simulink model "Test_newPR9July"  (R2022b)
settings: Solver=VariableStepAuto  StartTime=0.0  StopTime=25  RelTol=1e-3
values from neighbouring files (symbols this model uses):
  C_f = 0.000112315*9    (= 0.001010835)    [Main.m]    (also in PSO_2paras.m = swarm(i,2); PSO_filter_2paras.m = swarm(i,2)/10000; Primary_test1.m; Script_18June.m = 0.0112315)
  f_c = 50e3    (= 50000)    [Main.m]    (also in Primary_test1.m; Script_18June.m; Script_23June.m; Script_5thJune.m)
  k = -0.5    [Main.m]    (also in Primary_test1.m; Savedata.m = 0.2909; Script_18June.m = 0.5; Script_23June.m)
  K_h11 = 0    [Main.m]    (also in PSO_HC.m = swarm(i,4); Primary_test1.m; Script_18June.m; Script_23June.m)
  K_h13 = 0    [Main.m]    (also in Primary_test1.m; Script_18June.m; Script_23June.m; Script_5thJune.m)
  K_h5 = 0    [Main.m]    (also in PSO_HC.m = swarm(i,1); Primary_test1.m = 1; Script_18June.m; Script_23June.m)
  K_h7 = 0    [Main.m]    (also in PSO_HC.m = swarm(i,2); Primary_test1.m; Script_18June.m; Script_23June.m)
  K_h9 = 0    [Main.m]    (also in PSO_HC.m = swarm(i,3); Script_18June.m; Script_23June.m; Script_5thJune.m)
  ki_pr = 160    [Main.m]    (also in PSO.m = swarm(i,2); Primary_test1.m; Savedata.m = 422.4716; Script_18June.m = 150)
  kL = 1e-7    (= 1e-07)    [Main.m]    (also in Primary_test1.m; Script_18June.m; Script_23June.m; Script_5thJune.m)
  Kp_pr = 1.7    [Main.m]    (also in PSO.m = swarm(i,1); Primary_test1.m; Savedata.m = 0.9028; Script_18June.m = 1)
  L_f = 0.000659829*1.4    (= 0.0009237606)    [Main.m]    (also in PSO_2paras.m = swarm(i,1); PSO_filter_2paras.m = swarm(i,1); Primary_test1.m; Script_18June.m = 0.000295603392)
  L_in1 = 0.35e-3    (= 0.00035)    [Main.m]    (also in Primary_test1.m; Script_18June.m; Script_23June.m; Script_5thJune.m)
  L_in2 = 0.35e-3    (= 0.00035)    [Main.m]    (also in Primary_test1.m; Script_18June.m; Script_23June.m; Script_5thJune.m)
  LD_ref1 = 100e-6    (= 0.0001)    [Main.m]    (also in Primary_test1.m; Script_18June.m = 5e-05; Script_23June.m = 1e-05; Script_5thJune.m = 1e-05)
  lo_co = 0.1    [Main.m]    (also in Primary_test1.m; Script_18June.m; Script_23June.m; Script_5thJune.m)
  load_off = 28    [Main.m]    (also in Primary_test1.m = 2; Script_18June.m; Script_23June.m; Script_5thJune.m = 10)
  load_on = 0.21    [Main.m]    (also in Primary_test1.m = 1; Script_18June.m; Script_23June.m; Script_5thJune.m)
  m_p1 = 9.4e-5/droopDivide    (= 9.4e-06)    [Main.m]    (also in Primary_test1.m; Script_18June.m = 9.4e-05; Script_23June.m = 9.4e-05; Script_5thJune.m = 5e-05)
  m_p2 = 9.4e-5/droopDivide    (= 9.4e-06)    [Main.m]    (also in Primary_test1.m; Script_18June.m = 9.4e-05; Script_23June.m = 9.4e-05; Script_5thJune.m = 5e-05)
  m_p3 = 11.4e-5/droopDivide    (= 1.14e-05)    [Main.m]    (also in Primary_test1.m; Script_18June.m = 0.000114; Script_23June.m = 0.000114; Script_5thJune.m = 6.42857142857e-05)
  m_p4 = 11.4e-5/droopDivide    (= 1.14e-05)    [Main.m]    (also in Primary_test1.m; Script_18June.m = 0.000114; Script_23June.m = 0.000114; Script_5thJune.m = 6.42857142857e-05)
  n_q1 = 1.3e-3/droopDivide2    (= 6.5e-05)    [Main.m]    (also in Primary_test1.m; Script_18June.m; Script_23June.m; Script_5thJune.m = 0.2)
  n_q2 = 1.3e-3/droopDivide2    (= 6.5e-05)    [Main.m]    (also in Primary_test1.m; Script_18June.m; Script_23June.m; Script_5thJune.m = 0.2)
  n_q3 = 1.5e-3/droopDivide2    (= 7.5e-05)    [Main.m]    (also in Primary_test1.m; Script_18June.m; Script_23June.m; Script_5thJune.m = 0.257142857143)
  n_q4 = 1.5e-3/droopDivide2    (= 7.5e-05)    [Main.m]    (also in Primary_test1.m; Script_18June.m; Script_23June.m; Script_5thJune.m = 0.257142857143)
  PMW = V_nom/0.55    [Main.m]    (also in Primary_test1.m; Script_18June.m = V_nom/0.4; Script_23June.m; Script_5thJune.m = 220*sqrt(2))
  R_f = 0.35    [Main.m]    (also in PSO_filter_2paras.m = 10*L_f; Primary_test1.m; Savedata.m = 0.249593207053; Script_18June.m = 0.1)
  R_in1 = 0.03    [Main.m]    (also in Primary_test1.m; Script_18June.m; Script_23June.m; Script_5thJune.m)
  R_in2 = 0.03    [Main.m]    (also in Primary_test1.m; Script_18June.m; Script_23June.m; Script_5thJune.m)
  Ts = 10e-6    (= 1e-05)    [Main.m]    (also in Primary_test1.m; Script_18June.m; Script_23June.m; Script_5thJune.m)
  V_nom = 220*sqrt(2)    [Main.m]    (also in Primary_test1.m; Script_18June.m; Script_23June.m; Script_5thJune.m)
  Vdc = 600    [Main.m]    (also in Primary_test1.m; Script_18June.m; Script_23June.m; Script_5thJune.m)
  w_c_high = 2*pi*50    (= 314.159265359)    [Main.m]    (also in Primary_test1.m; Script_18June.m = 307.876080052; Script_23June.m; Script_5thJune.m = 307.876080052)
  w_nom = 2*pi*f    (= 314.159265359)    [Main.m]    (also in Primary_test1.m; Script_18June.m; Script_23June.m; Script_5thJune.m)
  wc_hc = 1    [Main.m]    (also in Primary_test1.m; Script_18June.m = 0.3; Script_23June.m; Script_5thJune.m = 0.3)
  wc_pr = 3    [Main.m]    (also in PSO.m = swarm(i,3); Primary_test1.m; Savedata.m = 1.36672; Script_18June.m = 1.5)
undefined symbols (not defined in the file or in its folder): i
libraries: eeGeneralControl x16, spsThreePhaseSeriesRLCBranchLib x15, spsThreePhaseVIMeasurementLib x12, spsabctodq0Lib x12, spsabctoAlphaBetaZeroLib x9, slpidlib x8, spsThreePhaseSeriesRLCLoadLib x6, spsThreePhaseBreakerLib x6, spsDCVoltageSourceLib x5, spsSeriesRLCBranchLib x5, spsTriangleGeneratorLib x4, spsTwoLevelConverterLib x4
(part 4 of 4)

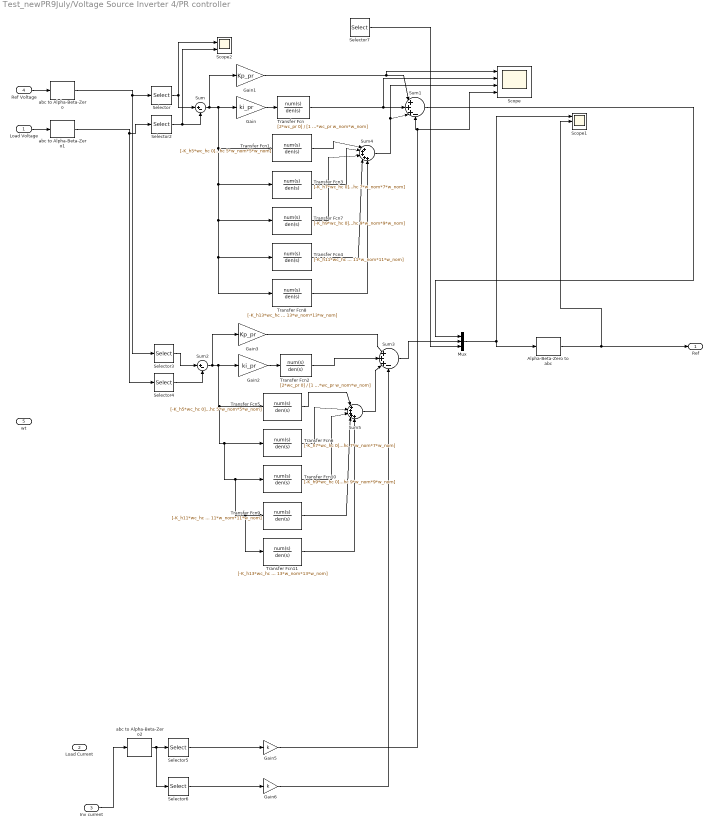
== system Test_newPR9July/Voltage Source Inverter 4/PR controller ==
  Load Voltage : Inport
  Load Current : Inport  Port=2
  Inv current : Inport  Port=3
  Ref Voltage : Inport  Port=4
  wt : Inport  Port=5
  Alpha-Beta-Zero to abc : spsAlphaBetaZerotoabcLib/Alpha-Beta-Zero to abc
      settings: LibrarySourceBlock=|
      | sps_lib/Control/Alpha-Beta-Zero
      | to abc
  Gain : Gain  Gain=ki_pr
  Gain1 : Gain  Gain=Kp_pr
  Gain2 : Gain  Gain=ki_pr
  Gain3 : Gain  Gain=Kp_pr
  Gain5 : Gain  Gain=k
  Gain6 : Gain  Gain=k
  Mux : Mux  Inputs=3
  Scope : Scope  NumInputPorts=4
  Scope1 : Scope  NumInputPorts=3
  Scope2 : Scope  NumInputPorts=2
  Selector : Selector  InputPortWidth=3  IndexOptions=Index vector (dialog)  Indices=[1]  OutputSizes=1
  Selector2 : Selector  InputPortWidth=3  IndexOptions=Index vector (dialog)  Indices=[1]  OutputSizes=1
  Selector3 : Selector  InputPortWidth=3  IndexOptions=Index vector (dialog)  Indices=[2]  OutputSizes=1
  Selector4 : Selector  InputPortWidth=3  IndexOptions=Index vector (dialog)  Indices=[2]  OutputSizes=1
  Selector5 : Selector  InputPortWidth=3  IndexOptions=Index vector (dialog)  Indices=[1]  OutputSizes=1
  Selector6 : Selector  InputPortWidth=3  IndexOptions=Index vector (dialog)  Indices=[2]  OutputSizes=1
  Selector7 : Selector  InputPortWidth=3  IndexOptions=Index vector (dialog)  Indices=[3]  OutputSizes=1
  Sum : Sum  Inputs=|+-
  Sum1 : Sum  Inputs=|+++-
  Sum2 : Sum  Inputs=|+-
  Sum3 : Sum  Inputs=|+++-
  Sum4 : Sum  Inputs=|+++++
  Sum5 : Sum  Inputs=|+++++
  Transfer Fcn : TransferFcn  Numerator=[2*wc_pr 0]  Denominator=[1 2*wc_pr*wc_pr w_nom*w_nom]
  Transfer Fcn1 : TransferFcn  Numerator=[-K_h5*wc_hc 0]  Denominator=[1 2*wc_hc 5*w_nom*5*w_nom]
  Transfer Fcn10 : TransferFcn  Numerator=[-K_h9*wc_hc 0]  Denominator=[1 2*wc_hc 9*w_nom*9*w_nom]
  Transfer Fcn11 : TransferFcn  Numerator=[-K_h13*wc_hc 0]  Denominator=[1 2*wc_hc 13*w_nom*13*w_nom]
  Transfer Fcn2 : TransferFcn  Numerator=[2*wc_pr 0]  Denominator=[1 2*wc_pr*wc_pr w_nom*w_nom]
  Transfer Fcn3 : TransferFcn  Numerator=[-K_h7*wc_hc 0]  Denominator=[1 2*wc_hc 7*w_nom*7*w_nom]
  Transfer Fcn4 : TransferFcn  Numerator=[-K_h11*wc_hc 0]  Denominator=[1 2*wc_hc 11*w_nom*11*w_nom]
  Transfer Fcn5 : TransferFcn  Numerator=[-K_h5*wc_hc 0]  Denominator=[1 2*wc_hc 5*w_nom*5*w_nom]
  Transfer Fcn6 : TransferFcn  Numerator=[-K_h7*wc_hc 0]  Denominator=[1 2*wc_hc 7*w_nom*7*w_nom]
  Transfer Fcn7 : TransferFcn  Numerator=[-K_h9*wc_hc 0]  Denominator=[1 2*wc_hc 9*w_nom*9*w_nom]
  Transfer Fcn8 : TransferFcn  Numerator=[-K_h13*wc_hc 0]  Denominator=[1 2*wc_hc 13*w_nom*13*w_nom]
  Transfer Fcn9 : TransferFcn  Numerator=[-K_h11*wc_hc 0]  Denominator=[1 2*wc_hc 11*w_nom*11*w_nom]
  abc to Alpha-Beta-Zero : spsabctoAlphaBetaZeroLib/abc to Alpha-Beta-Zero
  abc to Alpha-Beta-Zero1 : spsabctoAlphaBetaZeroLib/abc to Alpha-Beta-Zero
  abc to Alpha-Beta-Zero2 : spsabctoAlphaBetaZeroLib/abc to Alpha-Beta-Zero
  Ref : Outport
  wires:
  Ref Voltage/1 -> abc to Alpha-Beta-Zero/1
  Selector/1 -> Sum/1, Scope2/1
  Selector2/1 -> Sum/2, Scope2/2
  Sum/1 -> Gain1/1, Transfer Fcn8/1, Transfer Fcn4/1, Transfer Fcn7/1, Transfer Fcn3/1, Transfer Fcn1/1, Gain/1
  Gain/1 -> Transfer Fcn/1
  Gain1/1 -> Sum1/1, Scope/1
  Transfer Fcn/1 -> Scope/2, Sum1/2
  Sum2/1 -> Gain3/1, Transfer Fcn11/1, Transfer Fcn9/1, Transfer Fcn10/1, Transfer Fcn6/1, Transfer Fcn5/1, Gain2/1
  Selector3/1 -> Sum2/1
  Gain2/1 -> Transfer Fcn2/1
  Transfer Fcn2/1 -> Sum3/2
  Gain3/1 -> Sum3/1
  abc to Alpha-Beta-Zero2/1 -> Selector6/1, Selector5/1
  Sum1/1 -> Mux/1
  Sum3/1 -> Mux/2
  Mux/1 -> Alpha-Beta-Zero to abc/1, Scope1/1
  Inv current/1 -> abc to Alpha-Beta-Zero2/1
  Sum4/1 -> Sum1/3, Scope/3
  Transfer Fcn1/1 -> Sum4/1
  Transfer Fcn3/1 -> Sum4/2
  Transfer Fcn6/1 -> Sum5/2
  Selector4/1 -> Sum2/2
  Sum5/1 -> Sum3/3
  Transfer Fcn7/1 -> Sum4/3
  Transfer Fcn4/1 -> Sum4/4
  Transfer Fcn8/1 -> Sum4/5
  Transfer Fcn10/1 -> Sum5/3
  Transfer Fcn9/1 -> Sum5/4
  Transfer Fcn11/1 -> Sum5/5
  Selector6/1 -> Gain6/1
  Selector5/1 -> Gain5/1
  Transfer Fcn5/1 -> Sum5/1
  Selector7/1 -> Mux/3
  Gain5/1 -> Sum1/4, Scope/4
  Gain6/1 -> Sum3/4
  Load Voltage/1 -> abc to Alpha-Beta-Zero1/1
  abc to Alpha-Beta-Zero/1 -> Selector3/1, Selector/1
  abc to Alpha-Beta-Zero1/1 -> Selector4/1, Selector2/1
  Alpha-Beta-Zero to abc/1 -> Scope1/2, Ref/1

== system Test_newPR9July/Voltage Source Inverter 4/dq converter ==
  Vodq : Inport
  Iodq : Inport  Port=2
  Ildq : Inport  Port=3
  wt : Inport  Port=4
  Scope : Scope
  Scope1 : Scope
  Subsystem : Subsystem
  Subsystem1 : Subsystem
  Subsystem2 : Subsystem
  Vod : Outport
  Voq : Outport  Port=2
  Iod : Outport  Port=3
  Ioq : Outport  Port=4
  Ild : Outport  Port=5
  Ilq : Outport  Port=6
  wires:
  Subsystem/1(Out1) -> Scope/1, Vod/1  "Vod"
  Subsystem1/1(Out1) -> Iod/1  "Iod"
  Subsystem/2(Out2) -> Voq/1  "Voq"
  wt/1 -> Subsystem2/2(wt), Subsystem1/2(wt), Subsystem/2(wt)
  Subsystem1/2(Out2) -> Ioq/1  "Ioq"
  Iodq/1 -> Subsystem1/1(abc)
  Subsystem2/2(Out2) -> Ilq/1  "Ilq"
  Ildq/1 -> Subsystem2/1(abc)
  Vodq/1 -> Subsystem/1(abc)
  Subsystem2/1(Out1) -> Scope1/1, Ild/1  "Vod"

== system Test_newPR9July/Voltage Source Inverter 1/PLL_1p1/TienXuly ==
  v : Inport
  Gain : Gain  Gain=k
  Integrator : Integrator
  Integrator1 : Integrator
  Locthongthap : TransferFcn  Denominator=[1/fc2 1]
  Mux : Mux  Inputs=2
  Product : Product  RndMeth=Zero
  Product1 : Product  RndMeth=Zero
  Sum : Sum  Inputs=|+-
  Sum1 : Sum  Inputs=|+-
  Sum2 : Sum  Inputs=|+-
  v'-qv' : Scope
  wloc : Constant  Value=fc1*2*pi
  v' : Outport  VectorParamsAs1DForOutWhenUnconnected=off
  v'q : Outport  Port=2  VectorParamsAs1DForOutWhenUnconnected=off
  wires:
  Sum/1 -> Gain/1
  Gain/1 -> Sum1/1, Locthongthap/1
  Sum1/1 -> Product/1
  wloc/1 -> Product/2, Product1/1
  Product/1 -> Integrator/1
  Product1/1 -> Integrator1/1
  Integrator1/1 -> Sum1/2, Sum2/1
  Integrator/1 -> Product1/2, Sum/2, Mux/2, v'/1
  Locthongthap/1 -> Sum2/2
  v/1 -> Sum/1
  Sum2/1 -> v'q/1, Mux/1
  Mux/1 -> v'-qv'/1

== system Test_newPR9July/Voltage Source Inverter 1/PLL_1p1/apha-beta=>dq ==
  Theta : Inport
  Uapha : Inport  Port=2
  Ubeta : Inport  Port=3
  Mux : Mux  Inputs=3
  Tinhvd : Fcn  Expr=(u[2]*cos(u[1])+u[3]*sin(u[1]))
  Tinhvq : Fcn  Expr=(-u[2]*sin(u[1])+u[3]*cos(u[1]))
  vq : Outport  VectorParamsAs1DForOutWhenUnconnected=off
  vd : Outport  Port=2  VectorParamsAs1DForOutWhenUnconnected=off
  wires:
  Theta/1 -> Mux/1
  Uapha/1 -> Mux/2
  Ubeta/1 -> Mux/3
  Mux/1 -> Tinhvd/1, Tinhvq/1
  Tinhvd/1 -> vd/1
  Tinhvq/1 -> vq/1

== system Test_newPR9July/Voltage Source Inverter 1/PLL_1p2/TienXuly ==
  v : Inport
  Gain : Gain  Gain=k
  Integrator : Integrator
  Integrator1 : Integrator
  Locthongthap : TransferFcn  Denominator=[1/fc2 1]
  Mux : Mux  Inputs=2
  Product : Product  RndMeth=Zero
  Product1 : Product  RndMeth=Zero
  Sum : Sum  Inputs=|+-
  Sum1 : Sum  Inputs=|+-
  Sum2 : Sum  Inputs=|+-
  v'-qv' : Scope
  wloc : Constant  Value=fc1*2*pi
  v' : Outport  VectorParamsAs1DForOutWhenUnconnected=off
  v'q : Outport  Port=2  VectorParamsAs1DForOutWhenUnconnected=off
  wires:
  Sum/1 -> Gain/1
  Gain/1 -> Sum1/1, Locthongthap/1
  Sum1/1 -> Product/1
  wloc/1 -> Product/2, Product1/1
  Product/1 -> Integrator/1
  Product1/1 -> Integrator1/1
  Integrator1/1 -> Sum1/2, Sum2/1
  Integrator/1 -> Product1/2, Sum/2, Mux/2, v'/1
  Locthongthap/1 -> Sum2/2
  v/1 -> Sum/1
  Sum2/1 -> v'q/1, Mux/1
  Mux/1 -> v'-qv'/1

== system Test_newPR9July/Voltage Source Inverter 1/PLL_1p2/apha-beta=>dq ==
  Theta : Inport
  Uapha : Inport  Port=2
  Ubeta : Inport  Port=3
  Mux : Mux  Inputs=3
  Tinhvd : Fcn  Expr=(u[2]*cos(u[1])+u[3]*sin(u[1]))
  Tinhvq : Fcn  Expr=(-u[2]*sin(u[1])+u[3]*cos(u[1]))
  vq : Outport  VectorParamsAs1DForOutWhenUnconnected=off
  vd : Outport  Port=2  VectorParamsAs1DForOutWhenUnconnected=off
  wires:
  Theta/1 -> Mux/1
  Uapha/1 -> Mux/2
  Ubeta/1 -> Mux/3
  Mux/1 -> Tinhvd/1, Tinhvq/1
  Tinhvd/1 -> vd/1
  Tinhvq/1 -> vq/1

== system Test_newPR9July/Voltage Source Inverter 1/dq converter/Subsystem ==
  abc : Inport
  wt : Inport  Port=2
  Demux : Demux  Outputs=3
  abc to dq0 : spsabctodq0Lib/abc to dq0  Alignment=90 degrees behind phase A axis
  Out1 : Outport
  Out2 : Outport  Port=2
  wires:
  Demux/1 -> Out1/1
  abc to dq0/1 -> Demux/1
  wt/1 -> abc to dq0/2
  Demux/2 -> Out2/1
  abc/1 -> abc to dq0/1

== system Test_newPR9July/Voltage Source Inverter 1/dq converter/Subsystem1 ==
  abc : Inport
  wt : Inport  Port=2
  Demux : Demux  Outputs=3
  abc to dq0 : spsabctodq0Lib/abc to dq0  Alignment=90 degrees behind phase A axis
  Out1 : Outport
  Out2 : Outport  Port=2
  wires:
  Demux/1 -> Out1/1
  abc to dq0/1 -> Demux/1
  wt/1 -> abc to dq0/2
  Demux/2 -> Out2/1
  abc/1 -> abc to dq0/1

== system Test_newPR9July/Voltage Source Inverter 1/dq converter/Subsystem2 ==
  abc : Inport
  wt : Inport  Port=2
  Demux : Demux  Outputs=3
  abc to dq0 : spsabctodq0Lib/abc to dq0  Alignment=90 degrees behind phase A axis
  Out1 : Outport
  Out2 : Outport  Port=2
  wires:
  Demux/1 -> Out1/1
  abc to dq0/1 -> Demux/1
  wt/1 -> abc to dq0/2
  Demux/2 -> Out2/1
  abc/1 -> abc to dq0/1

== system Test_newPR9July/Voltage Source Inverter 2/PLL_1p1/TienXuly ==
  v : Inport
  Gain : Gain  Gain=k
  Integrator : Integrator
  Integrator1 : Integrator
  Locthongthap : TransferFcn  Denominator=[1/fc2 1]
  Mux : Mux  Inputs=2
  Product : Product  RndMeth=Zero
  Product1 : Product  RndMeth=Zero
  Sum : Sum  Inputs=|+-
  Sum1 : Sum  Inputs=|+-
  Sum2 : Sum  Inputs=|+-
  v'-qv' : Scope
  wloc : Constant  Value=fc1*2*pi
  v' : Outport  VectorParamsAs1DForOutWhenUnconnected=off
  v'q : Outport  Port=2  VectorParamsAs1DForOutWhenUnconnected=off
  wires:
  Sum/1 -> Gain/1
  Gain/1 -> Sum1/1, Locthongthap/1
  Sum1/1 -> Product/1
  wloc/1 -> Product/2, Product1/1
  Product/1 -> Integrator/1
  Product1/1 -> Integrator1/1
  Integrator1/1 -> Sum1/2, Sum2/1
  Integrator/1 -> Product1/2, Sum/2, Mux/2, v'/1
  Locthongthap/1 -> Sum2/2
  v/1 -> Sum/1
  Sum2/1 -> v'q/1, Mux/1
  Mux/1 -> v'-qv'/1

== system Test_newPR9July/Voltage Source Inverter 2/PLL_1p1/apha-beta=>dq ==
  Theta : Inport
  Uapha : Inport  Port=2
  Ubeta : Inport  Port=3
  Mux : Mux  Inputs=3
  Tinhvd : Fcn  Expr=(u[2]*cos(u[1])+u[3]*sin(u[1]))
  Tinhvq : Fcn  Expr=(-u[2]*sin(u[1])+u[3]*cos(u[1]))
  vq : Outport  VectorParamsAs1DForOutWhenUnconnected=off
  vd : Outport  Port=2  VectorParamsAs1DForOutWhenUnconnected=off
  wires:
  Theta/1 -> Mux/1
  Uapha/1 -> Mux/2
  Ubeta/1 -> Mux/3
  Mux/1 -> Tinhvd/1, Tinhvq/1
  Tinhvd/1 -> vd/1
  Tinhvq/1 -> vq/1

== system Test_newPR9July/Voltage Source Inverter 2/PLL_1p2/TienXuly ==
  v : Inport
  Gain : Gain  Gain=k
  Integrator : Integrator
  Integrator1 : Integrator
  Locthongthap : TransferFcn  Denominator=[1/fc2 1]
  Mux : Mux  Inputs=2
  Product : Product  RndMeth=Zero
  Product1 : Product  RndMeth=Zero
  Sum : Sum  Inputs=|+-
  Sum1 : Sum  Inputs=|+-
  Sum2 : Sum  Inputs=|+-
  v'-qv' : Scope
  wloc : Constant  Value=fc1*2*pi
  v' : Outport  VectorParamsAs1DForOutWhenUnconnected=off
  v'q : Outport  Port=2  VectorParamsAs1DForOutWhenUnconnected=off
  wires:
  Sum/1 -> Gain/1
  Gain/1 -> Sum1/1, Locthongthap/1
  Sum1/1 -> Product/1
  wloc/1 -> Product/2, Product1/1
  Product/1 -> Integrator/1
  Product1/1 -> Integrator1/1
  Integrator1/1 -> Sum1/2, Sum2/1
  Integrator/1 -> Product1/2, Sum/2, Mux/2, v'/1
  Locthongthap/1 -> Sum2/2
  v/1 -> Sum/1
  Sum2/1 -> v'q/1, Mux/1
  Mux/1 -> v'-qv'/1

== system Test_newPR9July/Voltage Source Inverter 2/PLL_1p2/apha-beta=>dq ==
  Theta : Inport
  Uapha : Inport  Port=2
  Ubeta : Inport  Port=3
  Mux : Mux  Inputs=3
  Tinhvd : Fcn  Expr=(u[2]*cos(u[1])+u[3]*sin(u[1]))
  Tinhvq : Fcn  Expr=(-u[2]*sin(u[1])+u[3]*cos(u[1]))
  vq : Outport  VectorParamsAs1DForOutWhenUnconnected=off
  vd : Outport  Port=2  VectorParamsAs1DForOutWhenUnconnected=off
  wires:
  Theta/1 -> Mux/1
  Uapha/1 -> Mux/2
  Ubeta/1 -> Mux/3
  Mux/1 -> Tinhvd/1, Tinhvq/1
  Tinhvd/1 -> vd/1
  Tinhvq/1 -> vq/1

== system Test_newPR9July/Voltage Source Inverter 2/dq converter/Subsystem ==
  abc : Inport
  wt : Inport  Port=2
  Demux : Demux  Outputs=3
  abc to dq0 : spsabctodq0Lib/abc to dq0  Alignment=90 degrees behind phase A axis
  Out1 : Outport
  Out2 : Outport  Port=2
  wires:
  Demux/1 -> Out1/1
  abc to dq0/1 -> Demux/1
  wt/1 -> abc to dq0/2
  Demux/2 -> Out2/1
  abc/1 -> abc to dq0/1

== system Test_newPR9July/Voltage Source Inverter 2/dq converter/Subsystem1 ==
  abc : Inport
  wt : Inport  Port=2
  Demux : Demux  Outputs=3
  abc to dq0 : spsabctodq0Lib/abc to dq0  Alignment=90 degrees behind phase A axis
  Out1 : Outport
  Out2 : Outport  Port=2
  wires:
  Demux/1 -> Out1/1
  abc to dq0/1 -> Demux/1
  wt/1 -> abc to dq0/2
  Demux/2 -> Out2/1
  abc/1 -> abc to dq0/1

== system Test_newPR9July/Voltage Source Inverter 2/dq converter/Subsystem2 ==
  abc : Inport
  wt : Inport  Port=2
  Demux : Demux  Outputs=3
  abc to dq0 : spsabctodq0Lib/abc to dq0  Alignment=90 degrees behind phase A axis
  Out1 : Outport
  Out2 : Outport  Port=2
  wires:
  Demux/1 -> Out1/1
  abc to dq0/1 -> Demux/1
  wt/1 -> abc to dq0/2
  Demux/2 -> Out2/1
  abc/1 -> abc to dq0/1

== system Test_newPR9July/Voltage Source Inverter 3/PLL_1p1/TienXuly ==
  v : Inport
  Gain : Gain  Gain=k
  Integrator : Integrator
  Integrator1 : Integrator
  Locthongthap : TransferFcn  Denominator=[1/fc2 1]
  Mux : Mux  Inputs=2
  Product : Product  RndMeth=Zero
  Product1 : Product  RndMeth=Zero
  Sum : Sum  Inputs=|+-
  Sum1 : Sum  Inputs=|+-
  Sum2 : Sum  Inputs=|+-
  v'-qv' : Scope
  wloc : Constant  Value=fc1*2*pi
  v' : Outport  VectorParamsAs1DForOutWhenUnconnected=off
  v'q : Outport  Port=2  VectorParamsAs1DForOutWhenUnconnected=off
  wires:
  Sum/1 -> Gain/1
  Gain/1 -> Sum1/1, Locthongthap/1
  Sum1/1 -> Product/1
  wloc/1 -> Product/2, Product1/1
  Product/1 -> Integrator/1
  Product1/1 -> Integrator1/1
  Integrator1/1 -> Sum1/2, Sum2/1
  Integrator/1 -> Product1/2, Sum/2, Mux/2, v'/1
  Locthongthap/1 -> Sum2/2
  v/1 -> Sum/1
  Sum2/1 -> v'q/1, Mux/1
  Mux/1 -> v'-qv'/1

== system Test_newPR9July/Voltage Source Inverter 3/PLL_1p1/apha-beta=>dq ==
  Theta : Inport
  Uapha : Inport  Port=2
  Ubeta : Inport  Port=3
  Mux : Mux  Inputs=3
  Tinhvd : Fcn  Expr=(u[2]*cos(u[1])+u[3]*sin(u[1]))
  Tinhvq : Fcn  Expr=(-u[2]*sin(u[1])+u[3]*cos(u[1]))
  vq : Outport  VectorParamsAs1DForOutWhenUnconnected=off
  vd : Outport  Port=2  VectorParamsAs1DForOutWhenUnconnected=off
  wires:
  Theta/1 -> Mux/1
  Uapha/1 -> Mux/2
  Ubeta/1 -> Mux/3
  Mux/1 -> Tinhvd/1, Tinhvq/1
  Tinhvd/1 -> vd/1
  Tinhvq/1 -> vq/1

== system Test_newPR9July/Voltage Source Inverter 3/PLL_1p2/TienXuly ==
  v : Inport
  Gain : Gain  Gain=k
  Integrator : Integrator
  Integrator1 : Integrator
  Locthongthap : TransferFcn  Denominator=[1/fc2 1]
  Mux : Mux  Inputs=2
  Product : Product  RndMeth=Zero
  Product1 : Product  RndMeth=Zero
  Sum : Sum  Inputs=|+-
  Sum1 : Sum  Inputs=|+-
  Sum2 : Sum  Inputs=|+-
  v'-qv' : Scope
  wloc : Constant  Value=fc1*2*pi
  v' : Outport  VectorParamsAs1DForOutWhenUnconnected=off
  v'q : Outport  Port=2  VectorParamsAs1DForOutWhenUnconnected=off
  wires:
  Sum/1 -> Gain/1
  Gain/1 -> Sum1/1, Locthongthap/1
  Sum1/1 -> Product/1
  wloc/1 -> Product/2, Product1/1
  Product/1 -> Integrator/1
  Product1/1 -> Integrator1/1
  Integrator1/1 -> Sum1/2, Sum2/1
  Integrator/1 -> Product1/2, Sum/2, Mux/2, v'/1
  Locthongthap/1 -> Sum2/2
  v/1 -> Sum/1
  Sum2/1 -> v'q/1, Mux/1
  Mux/1 -> v'-qv'/1

== system Test_newPR9July/Voltage Source Inverter 3/PLL_1p2/apha-beta=>dq ==
  Theta : Inport
  Uapha : Inport  Port=2
  Ubeta : Inport  Port=3
  Mux : Mux  Inputs=3
  Tinhvd : Fcn  Expr=(u[2]*cos(u[1])+u[3]*sin(u[1]))
  Tinhvq : Fcn  Expr=(-u[2]*sin(u[1])+u[3]*cos(u[1]))
  vq : Outport  VectorParamsAs1DForOutWhenUnconnected=off
  vd : Outport  Port=2  VectorParamsAs1DForOutWhenUnconnected=off
  wires:
  Theta/1 -> Mux/1
  Uapha/1 -> Mux/2
  Ubeta/1 -> Mux/3
  Mux/1 -> Tinhvd/1, Tinhvq/1
  Tinhvd/1 -> vd/1
  Tinhvq/1 -> vq/1

== system Test_newPR9July/Voltage Source Inverter 3/dq converter/Subsystem ==
  abc : Inport
  wt : Inport  Port=2
  Demux : Demux  Outputs=3
  abc to dq0 : spsabctodq0Lib/abc to dq0  Alignment=90 degrees behind phase A axis
  Out1 : Outport
  Out2 : Outport  Port=2
  wires:
  Demux/1 -> Out1/1
  abc to dq0/1 -> Demux/1
  wt/1 -> abc to dq0/2
  Demux/2 -> Out2/1
  abc/1 -> abc to dq0/1

== system Test_newPR9July/Voltage Source Inverter 3/dq converter/Subsystem1 ==
  abc : Inport
  wt : Inport  Port=2
  Demux : Demux  Outputs=3
  abc to dq0 : spsabctodq0Lib/abc to dq0  Alignment=90 degrees behind phase A axis
  Out1 : Outport
  Out2 : Outport  Port=2
  wires:
  Demux/1 -> Out1/1
  abc to dq0/1 -> Demux/1
  wt/1 -> abc to dq0/2
  Demux/2 -> Out2/1
  abc/1 -> abc to dq0/1

== system Test_newPR9July/Voltage Source Inverter 3/dq converter/Subsystem2 ==
  abc : Inport
  wt : Inport  Port=2
  Demux : Demux  Outputs=3
  abc to dq0 : spsabctodq0Lib/abc to dq0  Alignment=90 degrees behind phase A axis
  Out1 : Outport
  Out2 : Outport  Port=2
  wires:
  Demux/1 -> Out1/1
  abc to dq0/1 -> Demux/1
  wt/1 -> abc to dq0/2
  Demux/2 -> Out2/1
  abc/1 -> abc to dq0/1

== system Test_newPR9July/Voltage Source Inverter 4/PLL_1p1/TienXuly ==
  v : Inport
  Gain : Gain  Gain=k
  Integrator : Integrator
  Integrator1 : Integrator
  Locthongthap : TransferFcn  Denominator=[1/fc2 1]
  Mux : Mux  Inputs=2
  Product : Product  RndMeth=Zero
  Product1 : Product  RndMeth=Zero
  Sum : Sum  Inputs=|+-
  Sum1 : Sum  Inputs=|+-
  Sum2 : Sum  Inputs=|+-
  v'-qv' : Scope
  wloc : Constant  Value=fc1*2*pi
  v' : Outport  VectorParamsAs1DForOutWhenUnconnected=off
  v'q : Outport  Port=2  VectorParamsAs1DForOutWhenUnconnected=off
  wires:
  Sum/1 -> Gain/1
  Gain/1 -> Sum1/1, Locthongthap/1
  Sum1/1 -> Product/1
  wloc/1 -> Product/2, Product1/1
  Product/1 -> Integrator/1
  Product1/1 -> Integrator1/1
  Integrator1/1 -> Sum1/2, Sum2/1
  Integrator/1 -> Product1/2, Sum/2, Mux/2, v'/1
  Locthongthap/1 -> Sum2/2
  v/1 -> Sum/1
  Sum2/1 -> v'q/1, Mux/1
  Mux/1 -> v'-qv'/1

== system Test_newPR9July/Voltage Source Inverter 4/PLL_1p1/apha-beta=>dq ==
  Theta : Inport
  Uapha : Inport  Port=2
  Ubeta : Inport  Port=3
  Mux : Mux  Inputs=3
  Tinhvd : Fcn  Expr=(u[2]*cos(u[1])+u[3]*sin(u[1]))
  Tinhvq : Fcn  Expr=(-u[2]*sin(u[1])+u[3]*cos(u[1]))
  vq : Outport  VectorParamsAs1DForOutWhenUnconnected=off
  vd : Outport  Port=2  VectorParamsAs1DForOutWhenUnconnected=off
  wires:
  Theta/1 -> Mux/1
  Uapha/1 -> Mux/2
  Ubeta/1 -> Mux/3
  Mux/1 -> Tinhvd/1, Tinhvq/1
  Tinhvd/1 -> vd/1
  Tinhvq/1 -> vq/1

== system Test_newPR9July/Voltage Source Inverter 4/PLL_1p2/TienXuly ==
  v : Inport
  Gain : Gain  Gain=k
  Integrator : Integrator
  Integrator1 : Integrator
  Locthongthap : TransferFcn  Denominator=[1/fc2 1]
  Mux : Mux  Inputs=2
  Product : Product  RndMeth=Zero
  Product1 : Product  RndMeth=Zero
  Sum : Sum  Inputs=|+-
  Sum1 : Sum  Inputs=|+-
  Sum2 : Sum  Inputs=|+-
  v'-qv' : Scope
  wloc : Constant  Value=fc1*2*pi
  v' : Outport  VectorParamsAs1DForOutWhenUnconnected=off
  v'q : Outport  Port=2  VectorParamsAs1DForOutWhenUnconnected=off
  wires:
  Sum/1 -> Gain/1
  Gain/1 -> Sum1/1, Locthongthap/1
  Sum1/1 -> Product/1
  wloc/1 -> Product/2, Product1/1
  Product/1 -> Integrator/1
  Product1/1 -> Integrator1/1
  Integrator1/1 -> Sum1/2, Sum2/1
  Integrator/1 -> Product1/2, Sum/2, Mux/2, v'/1
  Locthongthap/1 -> Sum2/2
  v/1 -> Sum/1
  Sum2/1 -> v'q/1, Mux/1
  Mux/1 -> v'-qv'/1

== system Test_newPR9July/Voltage Source Inverter 4/PLL_1p2/apha-beta=>dq ==
  Theta : Inport
  Uapha : Inport  Port=2
  Ubeta : Inport  Port=3
  Mux : Mux  Inputs=3
  Tinhvd : Fcn  Expr=(u[2]*cos(u[1])+u[3]*sin(u[1]))
  Tinhvq : Fcn  Expr=(-u[2]*sin(u[1])+u[3]*cos(u[1]))
  vq : Outport  VectorParamsAs1DForOutWhenUnconnected=off
  vd : Outport  Port=2  VectorParamsAs1DForOutWhenUnconnected=off
  wires:
  Theta/1 -> Mux/1
  Uapha/1 -> Mux/2
  Ubeta/1 -> Mux/3
  Mux/1 -> Tinhvd/1, Tinhvq/1
  Tinhvd/1 -> vd/1
  Tinhvq/1 -> vq/1

== system Test_newPR9July/Voltage Source Inverter 4/dq converter/Subsystem ==
  abc : Inport
  wt : Inport  Port=2
  Demux : Demux  Outputs=3
  abc to dq0 : spsabctodq0Lib/abc to dq0  Alignment=90 degrees behind phase A axis
  Out1 : Outport
  Out2 : Outport  Port=2
  wires:
  Demux/1 -> Out1/1
  abc to dq0/1 -> Demux/1
  wt/1 -> abc to dq0/2
  Demux/2 -> Out2/1
  abc/1 -> abc to dq0/1

== system Test_newPR9July/Voltage Source Inverter 4/dq converter/Subsystem1 ==
  abc : Inport
  wt : Inport  Port=2
  Demux : Demux  Outputs=3
  abc to dq0 : spsabctodq0Lib/abc to dq0  Alignment=90 degrees behind phase A axis
  Out1 : Outport
  Out2 : Outport  Port=2
  wires:
  Demux/1 -> Out1/1
  abc to dq0/1 -> Demux/1
  wt/1 -> abc to dq0/2
  Demux/2 -> Out2/1
  abc/1 -> abc to dq0/1

== system Test_newPR9July/Voltage Source Inverter 4/dq converter/Subsystem2 ==
  abc : Inport
  wt : Inport  Port=2
  Demux : Demux  Outputs=3
  abc to dq0 : spsabctodq0Lib/abc to dq0  Alignment=90 degrees behind phase A axis
  Out1 : Outport
  Out2 : Outport  Port=2
  wires:
  Demux/1 -> Out1/1
  abc to dq0/1 -> Demux/1
  wt/1 -> abc to dq0/2
  Demux/2 -> Out2/1
  abc/1 -> abc to dq0/1
